simulink library "heli_2d_lib"  (Simulink 8.8)
settings: Solver=VariableStepAuto  StartTime=0.0  StopTime=10.0  RelTol=1e-3
values from neighbouring files (symbols this model uses):
  g = 9.81    [setup_heli_2d_configuration.m]
  J_eq_p = J_m_p + J_body_p + J_p + J_y    (= 0.0384309870395)    [setup_heli_2d_configuration.m]
  J_eq_y = J_m_y + J_body_y + J_p + J_y + J_shaft    (= 0.0431517259335)    [setup_heli_2d_configuration.m]
  K_pp = K_f_p * r_p    (= 0.20413345)    [setup_heli_2d_configuration.m]
  K_py = K_t_y / R_m_y    (= 0.0068125)    [setup_heli_2d_configuration.m]
  K_yp = K_t_p / R_m_p    (= 0.0219277108434)    [setup_heli_2d_configuration.m]
  K_yy = K_f_y * r_y    (= 0.071988045)    [setup_heli_2d_configuration.m]
  l_cm = ( (m_motor_p + m_shield ) * r_p +  (m_motor_y + m_shield ) * r_y ) / ( m_props )    (= 0.185670125995)    [setup_heli_2d_configuration.m]
  m_heli = 1.3872    [setup_heli_2d_configuration.m]
  SAT_INT_ERR_PITCH = 5    [setup_lab_heli_2d.m]
  SAT_INT_ERR_YAW = 5    [setup_lab_heli_2d.m]
  theta_0 = -40.5*pi/180    (= -0.706858347058)    [setup_lab_heli_2d.m]
  Tr_p = 1    [setup_lab_heli_2d.m]
  Tr_y = 1    [setup_lab_heli_2d.m]
  VMAX_UPM_P = 24    [setup_lab_heli_2d.m]
  VMAX_UPM_Y = 15    [setup_lab_heli_2d.m]
undefined symbols (not defined in the file or in its folder): B_p, B_y, K, Ki
libraries: heli_2d_lib x2
settings Model: SuppressorTable=22 serialization::archive 11 0 3 0 0 0 0 0  Creator=MLevis  LastModifiedBy=luy0a  ExtModeArmWhenConnect=off

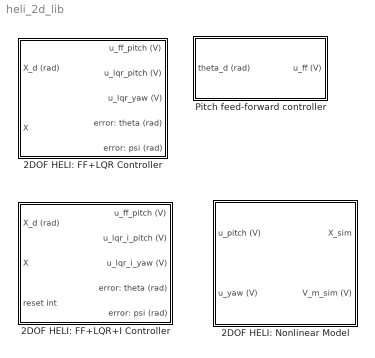
== system heli_2d_lib ==
  2DOF HELI: FF+LQR Controller : Subsystem
  2DOF HELI: FF+LQR+I Controller : Subsystem  AncestorBlock=heli_2d_lib/2DOF HELI: FF+LQR Controller
  2DOF HELI: Nonlinear Model : Subsystem  AncestorBlock=heli_2d_lib/2DOF Helicopter: Simple Nonlinear Model
  Pitch feed-forward controller : Subsystem  AncestorBlock=heli_2d_lib/2DOF HELI: FF+LQR+I Controller/Pitch feed-forward controller

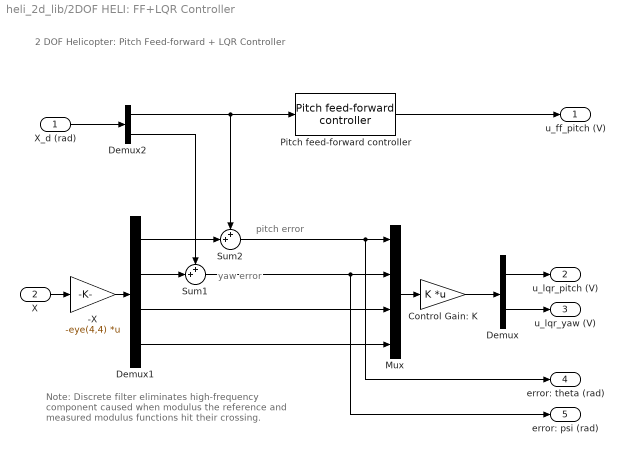
== system heli_2d_lib/2DOF HELI: FF+LQR Controller ==
  note: yaw error
  note: pitch error
  note: 2 DOF Helicopter:
      | Pitch Feed-forward + LQR Controller
  note: Note: Discrete filter eliminates high-frequency
      | component caused when modulus the reference
      | and measured modulus functions hit their crossing.
  X_d (rad) : Inport
  X : Inport  Port=2
  -X : Gain  Gain=-eye(4,4)  Multiplication=Matrix(K*u)
  Control Gain: K : Gain  Gain=K  Multiplication=Matrix(K*u)
  Demux : Demux  Outputs=2
  Demux1 : Demux
  Demux2 : Demux  Outputs=2
  Mux : Mux
  Pitch feed-forward controller : heli_2d_lib/Pitch feed-forward controller
  Sum1 : Sum  Inputs=++|
  Sum2 : Sum  Inputs=++|
  u_ff_pitch (V) : Outport
  u_lqr_pitch (V) : Outport  Port=2
  u_lqr_yaw (V) : Outport  Port=3
  error: theta (rad) : Outport  Port=4
  error: psi (rad) : Outport  Port=5
  wires:
  Pitch feed-forward controller/1 -> u_ff_pitch (V)/1
  Demux/1 -> u_lqr_pitch (V)/1
  Demux/2 -> u_lqr_yaw (V)/1
  Sum2/1 -> Mux/1, error: theta (rad)/1
  Demux1/1 -> Sum2/2
  X/1 -> -X/1
  -X/1 -> Demux1/1
  Control Gain: K/1 -> Demux/1
  Mux/1 -> Control Gain: K/1
  Demux1/3 -> Mux/3
  Demux1/4 -> Mux/4
  X_d (rad)/1 -> Demux2/1
  Demux1/2 -> Sum1/2
  Demux2/2 -> Sum1/1
  Demux2/1 -> Pitch feed-forward controller/1, Sum2/1
  Sum1/1 -> Mux/2, error: psi (rad)/1

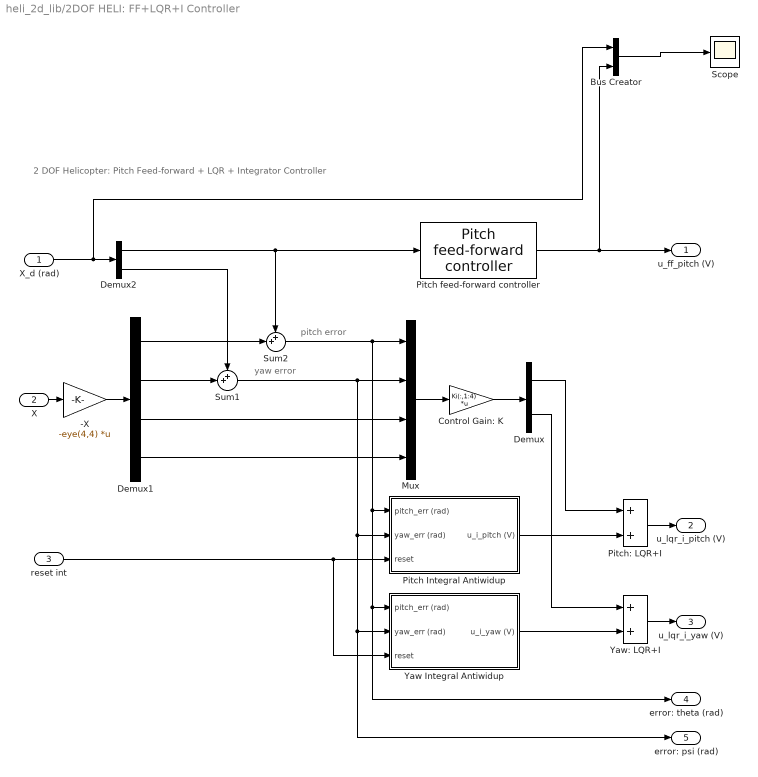
== system heli_2d_lib/2DOF HELI: FF+LQR+I Controller ==
  note: 2 DOF Helicopter:
      | Pitch Feed-forward + LQR + Integrator Controller
  note: pitch error
  note: yaw error
  X_d (rad) : Inport
  X : Inport  Port=2
  reset int : Inport  Port=3
  -X : Gain  Gain=-eye(4,4)  Multiplication=Matrix(K*u)
  Bus Creator : BusCreator  Inputs=2
  Control Gain: K : Gain  Gain=Ki(:,1:4)  Multiplication=Matrix(K*u)
  Demux : Demux  Outputs=2
  Demux1 : Demux
  Demux2 : Demux  Outputs=2
  Mux : Mux
  Pitch Integral Antiwidup : Subsystem  AncestorBlock=heli_2d_lib/2DOF HELI: FF+LQR+I Controller/Yaw Integral Antiwidup
  Pitch feed-forward controller : heli_2d_lib/Pitch feed-forward controller
  Pitch: LQR+I : Sum
  Scope : Scope
  Sum1 : Sum  Inputs=++|
  Sum2 : Sum  Inputs=++|
  Yaw Integral Antiwidup : Subsystem
  Yaw: LQR+I : Sum
  u_ff_pitch (V) : Outport
  u_lqr_i_pitch (V) : Outport  Port=2
  u_lqr_i_yaw (V) : Outport  Port=3
  error: theta (rad) : Outport  Port=4
  error: psi (rad) : Outport  Port=5
  wires:
  Demux1/4 -> Mux/4
  Demux1/3 -> Mux/3
  Mux/1 -> Control Gain: K/1
  Control Gain: K/1 -> Demux/1
  -X/1 -> Demux1/1
  Sum1/1 -> Mux/2, Pitch Integral Antiwidup/2(yaw_err (rad)), error: psi (rad)/1, Yaw Integral Antiwidup/2(yaw_err (rad))
  X/1 -> -X/1
  Demux1/1 -> Sum2/2
  Sum2/1 -> Pitch Integral Antiwidup/1(pitch_err (rad)), error: theta (rad)/1, Yaw Integral Antiwidup/1(pitch_err (rad)), Mux/1
  Pitch feed-forward controller/1 -> u_ff_pitch (V)/1, Bus Creator/2
  Pitch Integral Antiwidup/1(u_i_pitch (V)) -> Pitch: LQR+I/2
  Demux/1 -> Pitch: LQR+I/1
  Pitch: LQR+I/1 -> u_lqr_i_pitch (V)/1
  Yaw: LQR+I/1 -> u_lqr_i_yaw (V)/1
  Demux/2 -> Yaw: LQR+I/1
  Yaw Integral Antiwidup/1(u_i_yaw (V)) -> Yaw: LQR+I/2
  X_d (rad)/1 -> Bus Creator/1, Demux2/1
  Demux2/1 -> Pitch feed-forward controller/1, Sum2/1
  Demux2/2 -> Sum1/1
  Demux1/2 -> Sum1/2
  reset int/1 -> Yaw Integral Antiwidup/3(reset), Pitch Integral Antiwidup/3(reset)
  Bus Creator/1 -> Scope/1

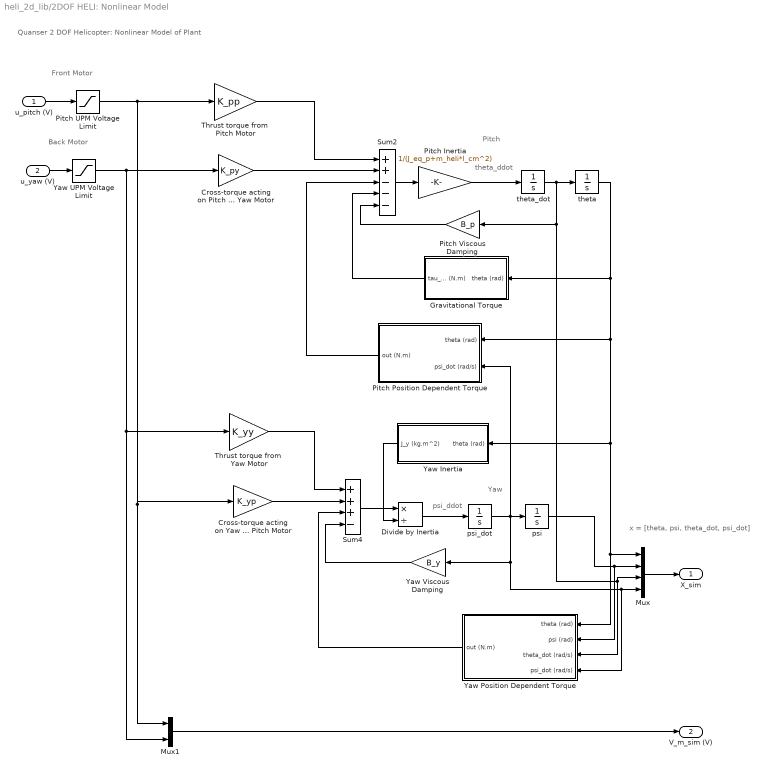
== system heli_2d_lib/2DOF HELI: Nonlinear Model ==
  note: Yaw
  note: Pitch
  note: psi_ddot
  note: theta_ddot
  note: Quanser 2 DOF Helicopter: Nonlinear Model of Plant
  note: x = [theta, psi, theta_dot, psi_dot]
  note: Front Motor
  note: Back Motor
  u_pitch (V) : Inport
  u_yaw (V) : Inport  Port=2
  Cross-torque acting on Pitch  from Yaw Motor : Gain  Gain=K_py
  Cross-torque acting on Yaw  from Pitch Motor : Gain  Gain=K_yp
  Divide by Inertia : Product  Inputs=*/
  Gravitational Torque : Subsystem
  Mux : Mux
  Mux1 : Mux  Inputs=2
  Pitch Inertia : Gain  Gain=1/(J_eq_p+m_heli*l_cm^2)
  Pitch Position Dependent Torque : Subsystem  AncestorBlock=heli_2d_lib/2DOF Helicopter: Nonlinear Model/Yaw Nonlinear Element
  Pitch UPM Voltage Limit : Saturate  UpperLimit=VMAX_UPM_P  LowerLimit=- VMAX_UPM_P
  Pitch Viscous Damping : Gain  Gain=B_p
  Sum2 : Sum  Inputs=++---
  Sum4 : Sum  Inputs=+++-
  Thrust torque from  Pitch Motor : Gain  Gain=K_pp
  Thrust torque from  Yaw Motor : Gain  Gain=K_yy
  Yaw Inertia : Subsystem
  Yaw Position Dependent Torque : Subsystem
  Yaw UPM Voltage Limit : Saturate  UpperLimit=VMAX_UPM_Y  LowerLimit=- VMAX_UPM_Y
  Yaw Viscous Damping : Gain  Gain=B_y
  psi : Integrator
  psi_dot : Integrator
  theta : Integrator  InitialCondition=theta_0  LimitOutput=on  UpperSaturationLimit=40.5*pi/180  LowerSaturationLimit=-40.5*pi/180
  theta_dot : Integrator
  X_sim : Outport
  V_m_sim (V) : Outport  Port=2
  wires:
  u_yaw (V)/1 -> Yaw UPM Voltage Limit/1
  u_pitch (V)/1 -> Pitch UPM Voltage Limit/1
  psi_dot/1 -> psi/1, Pitch Position Dependent Torque/2(psi_dot (rad/s)), Mux/4, Yaw Position Dependent Torque/4(psi_dot (rad/s)), Yaw Viscous Damping/1
  Cross-torque acting on Yaw  from Pitch Motor/1 -> Sum4/2
  Thrust torque from  Yaw Motor/1 -> Sum4/1
  theta_dot/1 -> theta/1, Mux/3, Yaw Position Dependent Torque/3(theta_dot (rad/s)), Pitch Viscous Damping/1
  Pitch Inertia/1 -> theta_dot/1
  Sum2/1 -> Pitch Inertia/1
  theta/1 -> Yaw Inertia/1(theta (rad)), Mux/1, Yaw Position Dependent Torque/1(theta (rad)), Pitch Position Dependent Torque/1(theta (rad)), Gravitational Torque/1(theta (rad))
  Mux/1 -> X_sim/1
  Pitch UPM Voltage Limit/1 -> Thrust torque from  Pitch Motor/1, Mux1/1, Cross-torque acting on Yaw  from Pitch Motor/1
  Yaw UPM Voltage Limit/1 -> Cross-torque acting on Pitch  from Yaw Motor/1, Mux1/2, Thrust torque from  Yaw Motor/1
  Mux1/1 -> V_m_sim (V)/1
  psi/1 -> Mux/2, Yaw Position Dependent Torque/2(psi (rad))
  Yaw Viscous Damping/1 -> Sum4/4
  Yaw Position Dependent Torque/1(out (N.m)) -> Sum4/3
  Sum4/1 -> Divide by Inertia/1
  Divide by Inertia/1 -> psi_dot/1
  Yaw Inertia/1(J_y (kg.m^2)) -> Divide by Inertia/2
  Thrust torque from  Pitch Motor/1 -> Sum2/1
  Cross-torque acting on Pitch  from Yaw Motor/1 -> Sum2/2
  Pitch Viscous Damping/1 -> Sum2/5
  Gravitational Torque/1(tau_g (N.m)) -> Sum2/4
  Pitch Position Dependent Torque/1(out (N.m)) -> Sum2/3

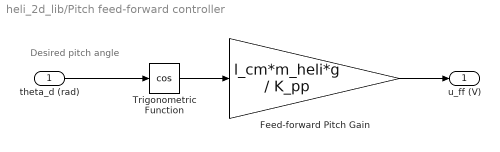
== system heli_2d_lib/Pitch feed-forward controller ==
  note: Desired pitch angle
  theta_d (rad) : Inport
  Feed-forward Pitch Gain : Gain  Gain=l_cm*m_heli*g / K_pp
  Trigonometric Function : Trigonometry  Operator=cos  OutputSignalType=real
  u_ff (V) : Outport
  wires:
  Trigonometric Function/1 -> Feed-forward Pitch Gain/1
  Feed-forward Pitch Gain/1 -> u_ff (V)/1
  theta_d (rad)/1 -> Trigonometric Function/1

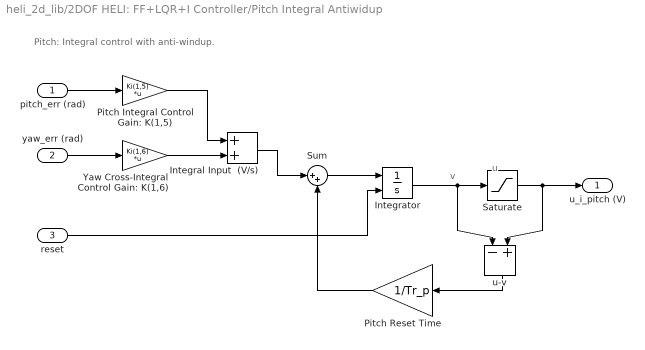
== system heli_2d_lib/2DOF HELI: FF+LQR+I Controller/Pitch Integral Antiwidup ==
  note: u
  note: v
  note: Pitch: Integral control with anti-windup.
  pitch_err (rad) : Inport
  yaw_err (rad) : Inport  Port=2
  reset : Inport  Port=3
  Integral Input  (V/s) : Sum
  Integrator : Integrator  ExternalReset=rising
  Pitch Integral Control Gain: K(1,5) : Gain  Gain=Ki(1,5)  Multiplication=Matrix(K*u)
  Pitch Reset Time : Gain  Gain=1/Tr_p
  Saturate : Saturate  UpperLimit=SAT_INT_ERR_PITCH  LowerLimit=-SAT_INT_ERR_PITCH
  Sum : Sum  Inputs=|++
  Yaw Cross-Integral Control Gain: K(1,6) : Gain  Gain=Ki(1,6)  Multiplication=Matrix(K*u)
  u-v : Sum  Inputs=-+
  u_i_pitch (V) : Outport
  wires:
  pitch_err (rad)/1 -> Pitch Integral Control Gain: K(1,5)/1
  Integrator/1 -> u-v/1, Saturate/1
  Saturate/1 -> u_i_pitch (V)/1, u-v/2
  u-v/1 -> Pitch Reset Time/1
  Sum/1 -> Integrator/1
  Pitch Reset Time/1 -> Sum/2
  reset/1 -> Integrator/2
  yaw_err (rad)/1 -> Yaw Cross-Integral Control Gain: K(1,6)/1
  Pitch Integral Control Gain: K(1,5)/1 -> Integral Input  (V/s)/1
  Yaw Cross-Integral Control Gain: K(1,6)/1 -> Integral Input  (V/s)/2
  Integral Input  (V/s)/1 -> Sum/1

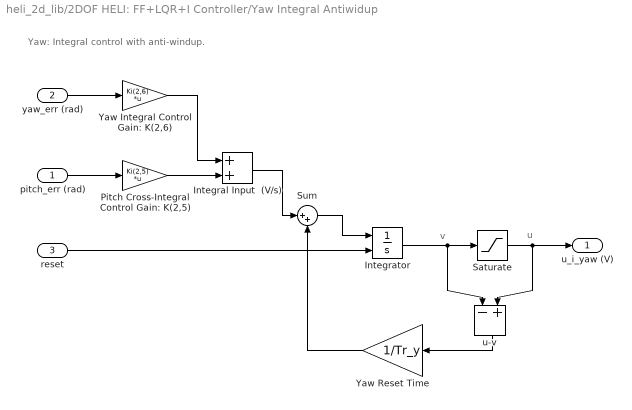
== system heli_2d_lib/2DOF HELI: FF+LQR+I Controller/Yaw Integral Antiwidup ==
  note: v
  note: u
  note: Yaw: Integral control with anti-windup.
  pitch_err (rad) : Inport
  yaw_err (rad) : Inport  Port=2
  reset : Inport  Port=3
  Integral Input  (V/s) : Sum
  Integrator : Integrator  ExternalReset=rising
  Pitch Cross-Integral Control Gain: K(2,5) : Gain  Gain=Ki(2,5)  Multiplication=Matrix(K*u)
  Saturate : Saturate  UpperLimit=SAT_INT_ERR_YAW  LowerLimit=-SAT_INT_ERR_YAW
  Sum : Sum  Inputs=|++
  Yaw Integral Control Gain: K(2,6) : Gain  Gain=Ki(2,6)  Multiplication=Matrix(K*u)
  Yaw Reset Time : Gain  Gain=1/Tr_y
  u-v : Sum  Inputs=-+
  u_i_yaw (V) : Outport
  wires:
  Yaw Reset Time/1 -> Sum/2
  Sum/1 -> Integrator/1
  u-v/1 -> Yaw Reset Time/1
  Saturate/1 -> u-v/2, u_i_yaw (V)/1
  Integrator/1 -> Saturate/1, u-v/1
  yaw_err (rad)/1 -> Yaw Integral Control Gain: K(2,6)/1
  reset/1 -> Integrator/2
  pitch_err (rad)/1 -> Pitch Cross-Integral Control Gain: K(2,5)/1
  Yaw Integral Control Gain: K(2,6)/1 -> Integral Input  (V/s)/1
  Pitch Cross-Integral Control Gain: K(2,5)/1 -> Integral Input  (V/s)/2
  Integral Input  (V/s)/1 -> Sum/1

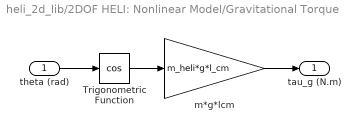
== system heli_2d_lib/2DOF HELI: Nonlinear Model/Gravitational Torque ==
  theta (rad) : Inport
  Trigonometric Function : Trigonometry  Operator=cos  OutputSignalType=real
  m*g*lcm : Gain  Gain=m_heli*g*l_cm
  tau_g (N.m) : Outport
  wires:
  Trigonometric Function/1 -> m*g*lcm/1
  theta (rad)/1 -> Trigonometric Function/1
  m*g*lcm/1 -> tau_g (N.m)/1

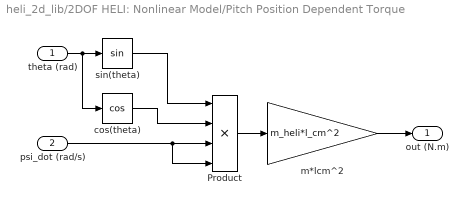
== system heli_2d_lib/2DOF HELI: Nonlinear Model/Pitch Position Dependent Torque ==
  theta (rad) : Inport
  psi_dot (rad/s) : Inport  Port=2
  Product : Product  Inputs=4  RndMeth=Zero
  cos(theta) : Trigonometry  Operator=cos  OutputSignalType=real
  m*lcm^2 : Gain  Gain=m_heli*l_cm^2
  sin(theta) : Trigonometry  OutputSignalType=real
  out (N.m) : Outport
  wires:
  m*lcm^2/1 -> out (N.m)/1
  cos(theta)/1 -> Product/2
  sin(theta)/1 -> Product/1
  Product/1 -> m*lcm^2/1
  theta (rad)/1 -> sin(theta)/1, cos(theta)/1
  psi_dot (rad/s)/1 -> Product/3, Product/4

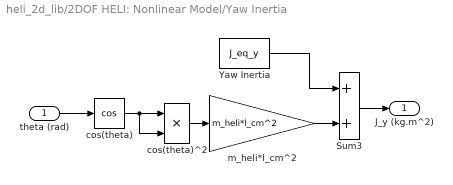
== system heli_2d_lib/2DOF HELI: Nonlinear Model/Yaw Inertia ==
  theta (rad) : Inport
  Sum3 : Sum
  Yaw Inertia : Constant  Value=J_eq_y
  cos(theta) : Trigonometry  Operator=cos  OutputSignalType=real
  cos(theta)^2 : Product  RndMeth=Zero
  m_heli*l_cm^2 : Gain  Gain=m_heli*l_cm^2
  J_y (kg.m^2) : Outport
  wires:
  cos(theta)^2/1 -> m_heli*l_cm^2/1
  Yaw Inertia/1 -> Sum3/1
  m_heli*l_cm^2/1 -> Sum3/2
  theta (rad)/1 -> cos(theta)/1
  Sum3/1 -> J_y (kg.m^2)/1
  cos(theta)/1 -> cos(theta)^2/1, cos(theta)^2/2

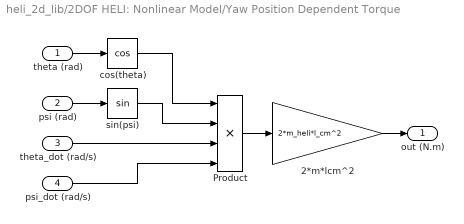
== system heli_2d_lib/2DOF HELI: Nonlinear Model/Yaw Position Dependent Torque ==
  theta (rad) : Inport
  psi (rad) : Inport  Port=2
  theta_dot (rad/s) : Inport  Port=3
  psi_dot (rad/s) : Inport  Port=4
  2*m*lcm^2 : Gain  Gain=2*m_heli*l_cm^2
  Product : Product  Inputs=4  RndMeth=Zero
  cos(theta) : Trigonometry  Operator=cos  OutputSignalType=real
  sin(psi) : Trigonometry  OutputSignalType=real
  out (N.m) : Outport
  wires:
  psi (rad)/1 -> sin(psi)/1
  theta (rad)/1 -> cos(theta)/1
  Product/1 -> 2*m*lcm^2/1
  cos(theta)/1 -> Product/1
  sin(psi)/1 -> Product/2
  theta_dot (rad/s)/1 -> Product/3
  psi_dot (rad/s)/1 -> Product/4
  2*m*lcm^2/1 -> out (N.m)/1
